simulink model "am_sys5"  (Simulink 3.00)
settings: Solver=ode45  StartTime=0.0  StopTime=999999  MaxStep=0.001  RelTol=1e-3  AbsTol=1e-3
settings Model: SaveTime=off  SaveOutput=off

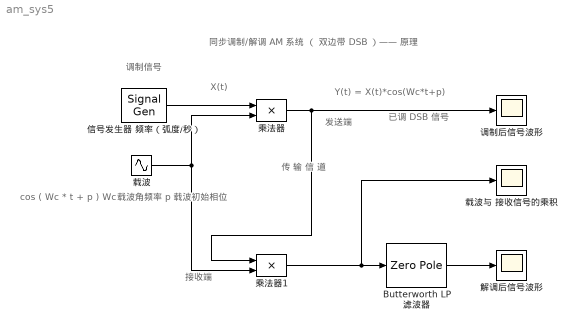
== system am_sys5 ==
  note: 传
      | 输
      | 信
      | 道
  note: 接收端
  note: Y(t) = X(t)*cos(Wc*t+p)
  note: X(t)
  note: 调制信号
  note: cos ( Wc * t + p )
      | Wc 载波角频率
      | p 载波初始相位
  note: 同步调制/解调 AM 系统 （ 双边带 DSB ）—— 原理
  note: 发送端
  note: 已调 DSB 信号
  Butterworth LP 滤波器 : ZeroPole  Zeros=z  Poles=p  Gain=k  mask(buttap){@1=10, @2=4}
      mask prompts: @1 "Cutoff frequency (rad/sec)"; @2 "Order"
      mask help:
      | Analog Butterworth low pass filter.
      |
      | (Requires Signal Processing Toolbox)
      mask init:
      | [z,p,k]=buttap(@2); z=@1*z; p=@1*p; k=real(prod(-p)); [num,den]=zp2tf(z,p,k); w=logspace(log10(@1/10),log10(10*@1),20); h=freqs(num,den,w);
      mask Help: Butterworth low pass filter using MATLAB's butter command.
      mask Display: plot(20*log10(w),20*log10(abs(h)))
  乘法器 : Product  Inputs=2  SaturateOnIntegerOverflow=on
      mask Type: 乘法器
      mask Description: 乘法器
      mask Display: plot([0 1],[1 0],[0 1],[0 1]);
  乘法器1 : Product  Inputs=2  SaturateOnIntegerOverflow=on
      mask Type: 乘法器
      mask Description: 乘法器
      mask Display: plot([0 1],[1 0],[0 1],[0 1]);
  调制后信号波形 : Scope
      settings: TimeRange=1.000000  YMin=-2  YMax=2  SaveToWorkspace=off  SaveName=ScopeData  DataFormat=Matrix
  解调后信号波形 : Scope
      settings: TimeRange=1.000000  YMin=-1  YMax=1  SaveToWorkspace=off  SaveName=ScopeData  DataFormat=Matrix
  信号发生器 频率（弧度/秒） : SignalGenerator  WaveForm=sine  Amplitude=1.000000  Frequency=10.000000  Units=rad/sec
  载波 : Sin  Amplitude=1  Frequency=100  Phase=0  SampleTime=0.001
  载波与 接收信号的乘积 : Scope
      settings: TimeRange=1.000000  YMin=-2  YMax=2  SaveToWorkspace=off  SaveName=ScopeData  DataFormat=Matrix
  wires:
  信号发生器 频率（弧度/秒）/1 -> 乘法器/1
  Butterworth LP 滤波器/1 -> 解调后信号波形/1
  载波/1 -> 乘法器/2, 乘法器1/2
  乘法器/1 -> 调制后信号波形/1, 乘法器1/1
  乘法器1/1 -> Butterworth LP 滤波器/1, 载波与 接收信号的乘积/1
